simulink model "lab2_2"  (R2020a)
settings: Solver=VariableStepAuto  StartTime=0.0  StopTime=10.0  RelTol=1e-10  AbsTol=1e-10
values from neighbouring files (symbols this model uses):
  g = 9.81    [lab2.m]
  km = 0.1    [lab2.m]
  La = 0.05    [lab2.m]
  M = 0.1    [lab2.m]
  Ra = 3    [lab2.m]
  ubar = ybar*Ra*sqrt(g*M/km)    [lab2.m]
  ybar = 0.1    [lab2.m]
libraries: cstblocks x1
settings Model: Creator=paulosga  LastModifiedBy=paulosga

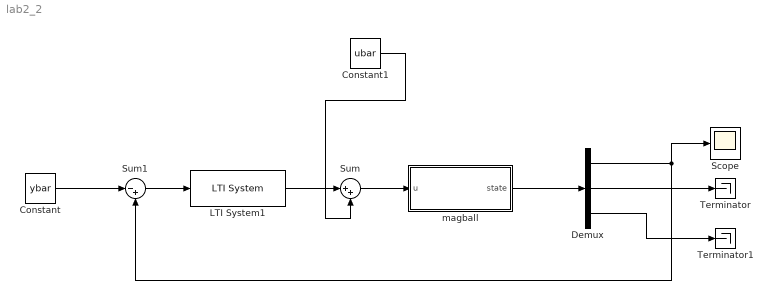
== system lab2_2 ==
  Constant : Constant  Value=ybar
  Constant1 : Constant  Value=ubar
  Demux : Demux  Outputs=3
  LTI System1 : cstblocks/LTI System  sys=CONTROLLER  IC=[]
  Scope : Scope
  Sum : Sum  Inputs=|++
  Sum1 : Sum  Inputs=|-+
  Terminator : Terminator
  Terminator1 : Terminator
  magball : Subsystem
  wires:
  LTI System1/1 -> Sum/1
  Demux/1 -> Sum1/2, Scope/1
  Demux/3 -> Terminator1/1
  Demux/2 -> Terminator/1
  magball/1(state) -> Demux/1
  Constant1/1 -> Sum/2
  Sum1/1 -> LTI System1/1
  Constant/1 -> Sum1/1
  Sum/1 -> magball/1(u)

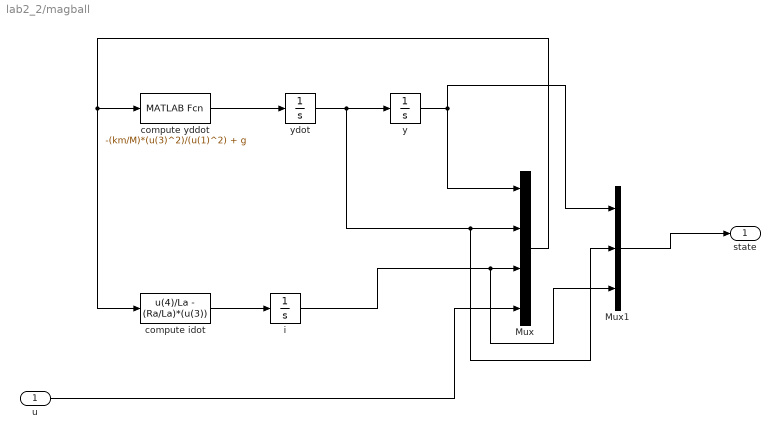
== system lab2_2/magball ==
  u : Inport
  Mux : Mux
  Mux1 : Mux  Inputs=3
  compute idot : MATLABFcn  MATLABFcn=u(4)/La - (Ra/La)*(u(3))
  compute yddot : MATLABFcn  MATLABFcn=-(km/M)*(u(3)^2)/(u(1)^2) + g
  i : Integrator
  y : Integrator
  ydot : Integrator
  state : Outport
  wires:
  ydot/1 -> Mux1/2, Mux/2, y/1
  compute yddot/1 -> ydot/1
  compute idot/1 -> i/1
  Mux1/1 -> state/1
  y/1 -> Mux1/1, Mux/1
  Mux/1 -> compute idot/1, compute yddot/1
  i/1 -> Mux1/3, Mux/3
  u/1 -> Mux/4
